simulink model "PubIfDecisionTOS_MDL"  (R2020b)
settings: configuration reference "DspaceConfig" (kept outside this file)
PostLoadFcn:
  | if any(exist('dsrtsu_mdlpostloadfcn', 'file') ~= 0), dsrtsu_mdlpostloadfcn('Execute', bdroot); end
InitFcn:
  | , if any(exist('dsmpb_private', 'file') ~= 0), dsmpb_private('dsmpb_mdlclblib', 'Init', bdroot); end,
undefined symbols (not defined in the file or in its folder): C_TOS_ACCEgoRAxletoFbumplength_m, C_TOS_ACCTargetFront_Flag, C_TOS_AEBJAPedObjDxThre_Val, C_TOS_AEBJAPedObjDyThre_Val, C_TOS_AEBJATargetSize_Val, C_TOS_AEBJAVehObjDxThre_Val, C_TOS_AEBJAVehObjDyThre_Val, C_TOS_AEBJuncPedTargetSize_Val, C_TOS_AEBLatObjDxThre_Val, C_TOS_AEBLatPedDyThre_Val, C_TOS_AEBLatTargetSize_Val, C_TOS_AEBLongTargetInEgoFront_Flag, C_TOS_axAbsGround_Parameter, C_TOS_CameraConfirmedFlag, C_TOS_CNsubjWidth, C_TOS_CurrentLaneCoreMinWidth_Val, C_TOS_CutInProb_Val_Zero, C_TOS_CutOutProb_Val_Zero, C_TOS_D2R_Val, C_TOS_DefaultValueObjectToCenterLine_dy, C_TOS_EgoCarWidth_Val, C_TOS_EgoDxRefPoint_m, C_TOS_EgoRAxletoFbumplength_m, C_TOS_HalfWidthVehicle_Con, C_TOS_HWA_CurrentLaneFlag, C_TOS_HWA_LeftLaneFlag, C_TOS_HWA_MovingDir_Vaild, C_TOS_HWA_MovState_Vaild, C_TOS_HWA_RightLaneFlag, C_TOS_LaneLineCourseErrorFront, C_TOS_LaneLineCourseErrorRear, C_TOS_MotorbikeDefaultWidth_m, C_TOS_NumberOfEffectiveTargets, C_TOS_Obj_Age_Val, C_TOS_Objdx_Constraint_Val, C_TOS_ObjectDefaultWidth_m, C_TOS_ObjInCurrentLane_Val, C_TOS_ObjInCurrentLaneValid, C_TOS_ObjInLeftLaneValid, C_TOS_ObjInRightLaneValid, C_TOS_ObjNotInCurrentLane_Val, C_TOS_ObjNotREElementType, C_TOS_ObjPredictDis_dy_ConstantVal_Zeros, C_TOS_ObjToCenterLine_ConstantVal_Zeros, C_TOS_OFMObjIDInvilad_Val, C_TOS_PIL_LatDisCons_Val_zero, C_TOS_PIL_ObjectCutInFlag_b, C_TOS_PIL_ObjectCutOutFlag_b, C_TOS_PIL_ObjLaneProb_al_Val, C_TOS_PP_ObjFusType_FC_Confirm_b, C_TOS_PP_ObjFusType_FC_FR_Confirm_b, C_TOS_PP_ObjFusType_FR_Confirm_b, C_TOS_RE_80BoolDefault_Val, C_TOS_RE_80Single181Default_Val, C_TOS_RE_80Single255Default_Val, C_TOS_RE_80Uint8Default_Val, C_TOS_RE_D2R, C_TOS_RE_D_180_Val, C_TOS_RE_InvalidObjectID_Val, C_TOS_RE_InvalidTargetChainDir_Val ... (+142)
libraries: simulink x1650, TOS_LIB x361, canfdmsglib x14
(part 9 of 69)

== system PubIfDecisionTOS_MDL/TOS_20201112/TOS_2012080320/PIL_1029/BoundaryCalculat/ObjectToCenterLine_dyc/RightLane ==
  CenterOfRightLane : Inport
  OFM_SignalVerification : Inport  Port=2
  Bus Selector : BusSelector  OutputSignals=TOS_OFMObjValid_Flag,Object_ID,Object_Age
  Bus Selector3 : BusSelector  OutputSignals=CenterLine01.PC0,CenterLine01.PC1,CenterLine01.PC2,CenterLine01.PC3,CenterLine01.dDisStart,CenterLine01.dDisEnd,CenterLine02.PC0,CenterLine02.PC1,CenterLine02.PC2,CenterLine02.PC3,CenterLine02.dDisStart,CenterLine02.dDisEnd,CenterLine03.PC0,CenterLine03.PC1,CenterLine03.PC2,CenterLine03.PC3,CenterLine03.dDisStart,CenterLine03.dDisEnd,CenterLine04.PC0,CenterLine04.PC1,CenterLine04.PC2,CenterLine04.PC3,CenterLine04.dDisStart,CenterLine04.dDisEnd,CenterLine05.PC0,CenterLine05.PC1,CenterLine05.PC2,CenterLine05.PC3,CenterLine05.dDisStart,CenterLine05.dDisEnd,CenterLine06.PC0,CenterLine06.PC1,CenterLine06.PC2,CenterLine06.PC3,CenterLine06.dDisStart,CenterLine06.dDisEnd
  Bus Selector4 : BusSelector  OutputSignals=TOS_OFMObjValid_Flag,Object_DY,Object_DX
  PIL_ObjectToCenterLine_dy_Filt : Subsystem
  RightCenterLine_dyc : Subsystem
  PIL_RightCenterLine_dyc : Outport
  PIL_RightCenterLine_dyc_Filt : Outport  Port=2
  wires:
  OFM_SignalVerification/1 -> [OFM_SignalVerification], Bus Selector4/1
  CenterOfRightLane/1 -> Bus Selector3/1
  Bus Selector3/34 -> RightCenterLine_dyc/37(line06_C3)  "<PC3>"
  Bus Selector3/35 -> RightCenterLine_dyc/38(line06_dDisStart)  "<dDisStart>"
  Bus Selector3/25 -> RightCenterLine_dyc/28(line05_C0)  "<PC0>"
  Bus Selector3/9 -> RightCenterLine_dyc/12(line02_C2)  "<PC2>"
  Bus Selector3/6 -> RightCenterLine_dyc/9(line01_dDisEnd)  "<dDisEnd>"
  Bus Selector3/22 -> RightCenterLine_dyc/25(line04_C3)  "<PC3>"
  Bus Selector3/31 -> RightCenterLine_dyc/34(line06_C0)  "<PC0>"
  Bus Selector3/16 -> RightCenterLine_dyc/19(line03_C3)  "<PC3>"
  Bus Selector3/8 -> RightCenterLine_dyc/11(line02_C1)  "<PC1>"
  Bus Selector4/1 -> RightCenterLine_dyc/1(TOS_OFMObjValid_Flag)  "<TOS_OFMObjValid_Flag>"
  Bus Selector3/33 -> RightCenterLine_dyc/36(line06_C2)  "<PC2>"
  Bus Selector3/10 -> RightCenterLine_dyc/13(line02_C3)  "<PC3>"
  Bus Selector3/14 -> RightCenterLine_dyc/17(line03_C1)  "<PC1>"
  Bus Selector3/1 -> RightCenterLine_dyc/4(line01_C0)  "<PC0>"
  Bus Selector3/28 -> RightCenterLine_dyc/31(line05_C3)  "<PC3>"
  Bus Selector3/32 -> RightCenterLine_dyc/35(line06_C1)  "<PC1>"
  Bus Selector3/27 -> RightCenterLine_dyc/30(line05_C2)  "<PC2>"
  Bus Selector3/20 -> RightCenterLine_dyc/23(line04_C1)  "<PC1>"
  Bus Selector3/30 -> RightCenterLine_dyc/33(line05_dDisEnd)  "<dDisEnd>"
  Bus Selector3/21 -> RightCenterLine_dyc/24(line04_C2)  "<PC2>"
  Bus Selector3/17 -> RightCenterLine_dyc/20(line03_dDisStart)  "<dDisStart>"
  Bus Selector3/26 -> RightCenterLine_dyc/29(line05_C1)  "<PC1>"
  Bus Selector3/11 -> RightCenterLine_dyc/14(line02_dDisStart)  "<dDisStart>"
  Bus Selector3/29 -> RightCenterLine_dyc/32(line05_dDisStart)  "<dDisStart>"
  Bus Selector3/24 -> RightCenterLine_dyc/27(line04_dDisEnd)  "<dDisEnd>"
  Bus Selector3/15 -> RightCenterLine_dyc/18(line03_C2)  "<PC2>"
  Bus Selector3/23 -> RightCenterLine_dyc/26(line04_dDisStart)  "<dDisStart>"
  Bus Selector4/2 -> RightCenterLine_dyc/2(Object_DY)  "<Object_DY>"
  Bus Selector3/13 -> RightCenterLine_dyc/16(line03_C0)  "<PC0>"
  Bus Selector3/19 -> RightCenterLine_dyc/22(line04_C0)  "<PC0>"
  Bus Selector3/36 -> RightCenterLine_dyc/39(line06_dDisEnd)  "<dDisEnd>"
  Bus Selector3/18 -> RightCenterLine_dyc/21(line03_dDisEnd)  "<dDisEnd>"
  Bus Selector3/12 -> RightCenterLine_dyc/15(line02_dDisEnd)  "<dDisEnd>"
  Bus Selector4/3 -> RightCenterLine_dyc/3(Object_DX)  "<Object_DX>"
  Bus Selector3/5 -> RightCenterLine_dyc/8(line01_dDisStart)  "<dDisStart>"
  Bus Selector3/7 -> RightCenterLine_dyc/10(line02_C0)  "<PC0>"
  Bus Selector3/4 -> RightCenterLine_dyc/7(line01_C3)  "<PC3>"
  Bus Selector3/3 -> RightCenterLine_dyc/6(line01_C2)  "<PC2>"
  Bus Selector3/2 -> RightCenterLine_dyc/5(line01_C1)  "<PC1>"
  Bus Selector/2 -> PIL_ObjectToCenterLine_dy_Filt/2(Object_ID)  "<Object_ID>"
  RightCenterLine_dyc/1(ObjectToCenterLine_dyc_RightLane) -> PIL_RightCenterLine_dyc/1, PIL_ObjectToCenterLine_dy_Filt/4(ObjectToCenterLine_dy)
  PIL_ObjectToCenterLine_dy_Filt/1(PIL_ObjectToCenterLine_dy_Filt) -> PIL_RightCenterLine_dyc_Filt/1
  Bus Selector/1 -> PIL_ObjectToCenterLine_dy_Filt/1(TOS_OFMObjValid_Flag)  "<TOS_OFMObjValid_Flag>"
  Bus Selector/3 -> PIL_ObjectToCenterLine_dy_Filt/3(Object_Age)  "<Object_Age>"
  [OFM_SignalVerification] -> Bus Selector/1

== system PubIfDecisionTOS_MDL/TOS_20201112/TOS_2012080320/PIL_1029/BoundaryCalculat/ObjectToCenterLine_dyc/SameLane ==
  Same_CenterLine : Inport
  OFM_SignalVerification : Inport  Port=2
  Bus Selector : BusSelector  OutputSignals=TOS_OFMObjValid_Flag,Object_ID,Object_Age
  Bus Selector3 : BusSelector  OutputSignals=CenterLine01.PC0,CenterLine01.PC1,CenterLine01.PC2,CenterLine01.PC3,CenterLine01.dDisStart,CenterLine01.dDisEnd,CenterLine02.PC0,CenterLine02.PC1,CenterLine02.PC2,CenterLine02.PC3,CenterLine02.dDisStart,CenterLine02.dDisEnd,CenterLine03.PC0,CenterLine03.PC1,CenterLine03.PC2,CenterLine03.PC3,CenterLine03.dDisStart,CenterLine03.dDisEnd,CenterLine04.PC0,CenterLine04.PC1,CenterLine04.PC2,CenterLine04.PC3,CenterLine04.dDisStart,CenterLine04.dDisEnd,CenterLine05.PC0,CenterLine05.PC1,CenterLine05.PC2,CenterLine05.PC3,CenterLine05.dDisStart,CenterLine05.dDisEnd,CenterLine06.PC0,CenterLine06.PC1,CenterLine06.PC2,CenterLine06.PC3,CenterLine06.dDisStart,CenterLine06.dDisEnd
  Bus Selector4 : BusSelector  OutputSignals=TOS_OFMObjValid_Flag,Object_DY,Object_DX
  PIL_ObjectToCenterLine_dy_Filt : Subsystem
  SameCenterLine_dyc : Subsystem
  PIL_SameCenterLine_dyc : Outport
  PIL_SameCenterLine_dyc_Filt : Outport  Port=2
  wires:
  Bus Selector3/2 -> SameCenterLine_dyc/5(line01_C1)  "<PC1>"
  Bus Selector3/3 -> SameCenterLine_dyc/6(line01_C2)  "<PC2>"
  Bus Selector3/4 -> SameCenterLine_dyc/7(line01_C3)  "<PC3>"
  Bus Selector3/7 -> SameCenterLine_dyc/10(line02_C0)  "<PC0>"
  Bus Selector3/5 -> SameCenterLine_dyc/8(line01_dDisStart)  "<dDisStart>"
  Bus Selector4/3 -> SameCenterLine_dyc/3(Object_DX)  "<Object_DX>"
  Bus Selector3/12 -> SameCenterLine_dyc/15(line02_dDisEnd)  "<dDisEnd>"
  Bus Selector3/18 -> SameCenterLine_dyc/21(line03_dDisEnd)  "<dDisEnd>"
  Bus Selector3/36 -> SameCenterLine_dyc/39(line06_dDisEnd)  "<dDisEnd>"
  Bus Selector3/19 -> SameCenterLine_dyc/22(line04_C0)  "<PC0>"
  Bus Selector3/13 -> SameCenterLine_dyc/16(line03_C0)  "<PC0>"
  Bus Selector4/2 -> SameCenterLine_dyc/2(Object_DY)  "<Object_DY>"
  Bus Selector3/23 -> SameCenterLine_dyc/26(line04_dDisStart)  "<dDisStart>"
  Bus Selector3/15 -> SameCenterLine_dyc/18(line03_C2)  "<PC2>"
  Bus Selector3/24 -> SameCenterLine_dyc/27(line04_dDisEnd)  "<dDisEnd>"
  Bus Selector3/29 -> SameCenterLine_dyc/32(line05_dDisStart)  "<dDisStart>"
  Bus Selector3/11 -> SameCenterLine_dyc/14(line02_dDisStart)  "<dDisStart>"
  Bus Selector3/26 -> SameCenterLine_dyc/29(line05_C1)  "<PC1>"
  Bus Selector3/17 -> SameCenterLine_dyc/20(line03_dDisStart)  "<dDisStart>"
  Bus Selector3/21 -> SameCenterLine_dyc/24(line04_C2)  "<PC2>"
  Bus Selector3/30 -> SameCenterLine_dyc/33(line05_dDisEnd)  "<dDisEnd>"
  Bus Selector3/20 -> SameCenterLine_dyc/23(line04_C1)  "<PC1>"
  Bus Selector3/27 -> SameCenterLine_dyc/30(line05_C2)  "<PC2>"
  Bus Selector3/32 -> SameCenterLine_dyc/35(line06_C1)  "<PC1>"
  Bus Selector3/28 -> SameCenterLine_dyc/31(line05_C3)  "<PC3>"
  Bus Selector3/1 -> SameCenterLine_dyc/4(line01_C0)  "<PC0>"
  Bus Selector3/14 -> SameCenterLine_dyc/17(line03_C1)  "<PC1>"
  Bus Selector3/10 -> SameCenterLine_dyc/13(line02_C3)  "<PC3>"
  Bus Selector3/33 -> SameCenterLine_dyc/36(line06_C2)  "<PC2>"
  Bus Selector4/1 -> SameCenterLine_dyc/1(TOS_OFMObjValid_Flag)  "<TOS_OFMObjValid_Flag>"
  Bus Selector3/8 -> SameCenterLine_dyc/11(line02_C1)  "<PC1>"
  Bus Selector3/16 -> SameCenterLine_dyc/19(line03_C3)  "<PC3>"
  Bus Selector3/31 -> SameCenterLine_dyc/34(line06_C0)  "<PC0>"
  Bus Selector3/22 -> SameCenterLine_dyc/25(line04_C3)  "<PC3>"
  Bus Selector3/6 -> SameCenterLine_dyc/9(line01_dDisEnd)  "<dDisEnd>"
  Bus Selector3/9 -> SameCenterLine_dyc/12(line02_C2)  "<PC2>"
  Bus Selector3/25 -> SameCenterLine_dyc/28(line05_C0)  "<PC0>"
  Bus Selector3/35 -> SameCenterLine_dyc/38(line06_dDisStart)  "<dDisStart>"
  Bus Selector3/34 -> SameCenterLine_dyc/37(line06_C3)  "<PC3>"
  Same_CenterLine/1 -> Bus Selector3/1
  OFM_SignalVerification/1 -> [OFM_SignalVerification], Bus Selector4/1
  Bus Selector/2 -> PIL_ObjectToCenterLine_dy_Filt/2(Object_ID)  "<Object_ID>"
  SameCenterLine_dyc/1(SameCenterLine_dyc) -> PIL_SameCenterLine_dyc/1, PIL_ObjectToCenterLine_dy_Filt/4(ObjectToCenterLine_dy)
  PIL_ObjectToCenterLine_dy_Filt/1(PIL_ObjectToCenterLine_dy_Filt) -> PIL_SameCenterLine_dyc_Filt/1
  Bus Selector/1 -> PIL_ObjectToCenterLine_dy_Filt/1(TOS_OFMObjValid_Flag)  "<TOS_OFMObjValid_Flag>"
  Bus Selector/3 -> PIL_ObjectToCenterLine_dy_Filt/3(Object_Age)  "<Object_Age>"
  [OFM_SignalVerification] -> Bus Selector/1

== system PubIfDecisionTOS_MDL/TOS_20201112/TOS_2012080320/PIL_1029/ObjCutInOut_Prob/ObjectCutIn/CutInProb_Calculate ==
  TOS_OFMObjValid_Flag : Inport  Partition=on  PartitionDimension=1  PartitionWidth=1  PartitionOffset=0
  Object_Width : Inport  Port=2  OutDataTypeStr=single  Partition=on  PartitionDimension=1  PartitionWidth=1  PartitionOffset=0
  Object_DX : Inport  Port=3  OutDataTypeStr=single  Partition=on  PartitionDimension=1  PartitionWidth=1  PartitionOffset=0
  Object_DY : Inport  Port=4  OutDataTypeStr=single  Partition=on  PartitionDimension=1  PartitionWidth=1  PartitionOffset=0
  Object_Age : Inport  Port=5  OutDataTypeStr=uint16  Partition=on  PartitionDimension=1  PartitionWidth=1  PartitionOffset=0
  Object_Type : Inport  Port=6  Partition=on  PartitionDimension=1  PartitionWidth=1  PartitionOffset=0
  PP_ObjectToCenterLine_dy : Inport  Port=7  OutDataTypeStr=single  Partition=on  PartitionDimension=1  PartitionWidth=1  PartitionOffset=0
  PP_ObjectToCenterLine_vyc : Inport  Port=8  OutDataTypeStr=single  Partition=on  PartitionDimension=1  PartitionWidth=1  PartitionOffset=0
  PIL_ObjectToCenterLine_dy_Filt : Inport  Port=9  OutDataTypeStr=single  Partition=on  PartitionDimension=1  PartitionWidth=1  PartitionOffset=0
  PP_CurrentLaneWidth : Inport  Port=10
  Compare To Constant : simulink/Logic and Bit Operations/Compare To Constant  relop===  const=C_TOS_OFMObjIDInvilad_Val  OutDataTypeStr=boolean
      settings: AttributesFormatString=C_TOS_OFMObjIDInvilad_Val = 0
  CutInProb_CalculateDefault : Subsystem  TreatAsAtomicUnit=on
  CutInProb_Calculate_ : Subsystem
  For Each : ForEach  DisableCoverage=on
  If : If  IfExpression=u1 ~= 0
  Merge{,1..4} (5 alike) : Merge
  PIL_CutInPredictTime_ObserVale : Outport  OutDataTypeStr=single  ConcatenationDimension=1
  PIL_CutInPredictTime_dxConstraint_ObserVale : Outport  Port=2  OutDataTypeStr=single  ConcatenationDimension=1
  PIL_CutInPredictDis_dy_ObjWidthConstraint_ObserVale : Outport  Port=3  ConcatenationDimension=1
  PIL_ObjectCutinMindFlg_ObserVale : Outport  Port=4  OutDataTypeStr=boolean  ConcatenationDimension=1
  CutInProb_Calculate : Outport  Port=5  ConcatenationDimension=1
  wires:
  Object_Width/1 -> CutInProb_Calculate_/1(Object_Width)  "Object_Width"
  Object_DX/1 -> CutInProb_Calculate_/2(Object_DX)  "Object_DX"
  Object_DY/1 -> CutInProb_Calculate_/3(Object_DY)  "Object_DY"
  Object_Age/1 -> CutInProb_Calculate_/4(Object_Age)  "Object_Age"
  Object_Type/1 -> CutInProb_Calculate_/5(Object_Type)  "Object_Type"
  PP_ObjectToCenterLine_dy/1 -> CutInProb_Calculate_/6(PP_ObjectToCenterLine_dy)  "PP_ObjectToCenterLine_dy"
  PP_ObjectToCenterLine_vyc/1 -> CutInProb_Calculate_/7(PP_ObjectToCenterLine_vyc)  "PP_ObjectToCenterLine_vyc"
  PIL_ObjectToCenterLine_dy_Filt/1 -> CutInProb_Calculate_/8(PIL_ObjectToCenterLine_dy_Filt)  "PIL_ObjectToCenterLine_dy_Filt"
  PP_CurrentLaneWidth/1 -> CutInProb_Calculate_/9(PP_CurrentLaneWidth)  "CurrentLaneWidth"
  TOS_OFMObjValid_Flag/1 -> Compare To Constant/1
  If/2 -> CutInProb_Calculate_/Action
  Compare To Constant/1 -> If/1
  If/1 -> CutInProb_CalculateDefault/Action
  CutInProb_Calculate_/1(PIL_CutInPredictTime_ObserVale) -> Merge/2
  CutInProb_Calculate_/2(PIL_CutInPredictTime_dxConstraint_ObserVale) -> Merge1/2
  CutInProb_Calculate_/3(PIL_CutInPredictDis_dy_ObjWidthConstraint_ObserVale) -> Merge2/2
  CutInProb_Calculate_/4(PIL_ObjectCutinMindFlg_ObserVale) -> Merge3/2
  CutInProb_Calculate_/5(CutInProb_Calculate) -> Merge4/2
  CutInProb_CalculateDefault/1(PIL_CutInPredictTime_ObserVale) -> Merge/1
  CutInProb_CalculateDefault/2(PIL_CutInPredictTime_dxConstraint_ObserVale) -> Merge1/1
  CutInProb_CalculateDefault/3(PIL_CutInPredictDis_dy_ObjWidthConstraint_ObserVale) -> Merge2/1
  CutInProb_CalculateDefault/4(PIL_ObjectCutinMindFlg_ObserVale) -> Merge3/1
  CutInProb_CalculateDefault/5(CutInProb_Calculate) -> Merge4/1
  Merge/1 -> PIL_CutInPredictTime_ObserVale/1
  Merge1/1 -> PIL_CutInPredictTime_dxConstraint_ObserVale/1
  Merge2/1 -> PIL_CutInPredictDis_dy_ObjWidthConstraint_ObserVale/1
  Merge3/1 -> PIL_ObjectCutinMindFlg_ObserVale/1
  Merge4/1 -> CutInProb_Calculate/1

== system PubIfDecisionTOS_MDL/TOS_20201112/TOS_2012080320/PIL_1029/ObjCutInOut_Prob/ObjectCutIn/CutInProb_Pluse ==
  CutInProb_Pluse_K1 : Inport  OutDataTypeStr=single  Partition=on  PartitionDimension=1  PartitionWidth=1  PartitionOffset=0
  CutInProb_ScopeConstraint : Inport  Port=2  OutDataTypeStr=single  Partition=on  PartitionDimension=1  PartitionWidth=1  PartitionOffset=0
  Object_Dx : Inport  Port=3  OutDataTypeStr=single  Partition=on  PartitionDimension=1  PartitionWidth=1  PartitionOffset=0
  TOS_OFMObjValid_Flag : Inport  Port=4  Partition=on  PartitionDimension=1  PartitionWidth=1  PartitionOffset=0
  Object_MovingState : Inport  Port=5  Partition=on  PartitionDimension=1  PartitionWidth=1  PartitionOffset=0
  Compare To Constant1 : simulink/Logic and Bit Operations/Compare To Constant  relop=~=  const=C_TOS_OFMObjIDInvilad_Val  OutDataTypeStr=boolean
      settings: AttributesFormatString=C_TOS_OFMObjIDInvilad_Val = 0
  Compare To Constant6 : simulink/Logic and Bit Operations/Compare To Constant  relop===  const=OFM_OBJ_MOVINGSTATE_E.MOVING  OutDataTypeStr=boolean
      settings: AttributesFormatString=OFM_OBJ_MOVINGSTATE_E.MOVING = 2
  CutInProb_Pluse : Subsystem
  CutInProb_PluseDefault : Subsystem  TreatAsAtomicUnit=on
  Data Type Conversion1 : DataTypeConversion  OutDataTypeStr=Enum: OFM_OBJ_MOVINGSTATE_E
  For Each : ForEach  DisableCoverage=on
  If1 : If  IfExpression=u1 == 1
  Logical Operator2 : Logic  AllPortsSameDT=off  OutDataTypeStr=boolean
  Merge : Merge
  Merge1 : Merge
  PIL_CutInProb_Pluse : Outport  OutDataTypeStr=single  ConcatenationDimension=1
  PIL_ObjectCutInFlag : Outport  Port=2  ConcatenationDimension=1
  wires:
  CutInProb_Pluse/2(PIL_ObjectCutInFlag) -> Merge1/1
  CutInProb_Pluse/1(PIL_CutInProb_Pluse) -> Merge/1
  CutInProb_PluseDefault/2(PIL_ObjectCutInFlag) -> Merge1/2
  CutInProb_PluseDefault/1(PIL_CutInProb_Pluse) -> Merge/2
  Data Type Conversion1/1 -> Compare To Constant6/1
  Compare To Constant6/1 -> Logical Operator2/2
  TOS_OFMObjValid_Flag/1 -> Compare To Constant1/1
  Object_MovingState/1 -> Data Type Conversion1/1
  Logical Operator2/1 -> If1/1
  Compare To Constant1/1 -> Logical Operator2/1
  CutInProb_Pluse_K1/1 -> CutInProb_Pluse/1(CutInProb_Pluse_K1)
  CutInProb_ScopeConstraint/1 -> CutInProb_Pluse/2(CutInProb_ScopeConstraint)
  Object_Dx/1 -> CutInProb_Pluse/3(Object_Dx)
  If1/2 -> CutInProb_PluseDefault/Action
  If1/1 -> CutInProb_Pluse/Action
  Merge/1 -> PIL_CutInProb_Pluse/1
  Merge1/1 -> PIL_ObjectCutInFlag/1

== system PubIfDecisionTOS_MDL/TOS_20201112/TOS_2012080320/PIL_1029/ObjCutInOut_Prob/ObjectCutOut/CutOutProb_Calculate ==
  TOS_OFMObjValid_Flag : Inport  Partition=on  PartitionDimension=1  PartitionWidth=1  PartitionOffset=0
  Object_Width : Inport  Port=2  Partition=on  PartitionDimension=1  PartitionWidth=1  PartitionOffset=0
  Object_DX : Inport  Port=3  Partition=on  PartitionDimension=1  PartitionWidth=1  PartitionOffset=0
  Object_DY : Inport  Port=4  Partition=on  PartitionDimension=1  PartitionWidth=1  PartitionOffset=0
  Object_Age : Inport  Port=5  Partition=on  PartitionDimension=1  PartitionWidth=1  PartitionOffset=0
  Object_Type : Inport  Port=6  Partition=on  PartitionDimension=1  PartitionWidth=1  PartitionOffset=0
  PP_ObjectToCenterLine_dy : Inport  Port=7  Partition=on  PartitionDimension=1  PartitionWidth=1  PartitionOffset=0
  PP_ObjectToCenterLine_vyc : Inport  Port=8  Partition=on  PartitionDimension=1  PartitionWidth=1  PartitionOffset=0
  PIL_ObjectToCenterLine_dy_Filt : Inport  Port=9  Partition=on  PartitionDimension=1  PartitionWidth=1  PartitionOffset=0
  Object_VY : Inport  Port=10  Partition=on  PartitionDimension=1  PartitionWidth=1  PartitionOffset=0
  Compare To Constant : simulink/Logic and Bit Operations/Compare To Constant  relop===  const=C_TOS_OFMObjIDInvilad_Val  OutDataTypeStr=boolean
      settings: AttributesFormatString=C_TOS_OFMObjIDInvilad_Val = 0
  CutOutProb_Calculate : Subsystem
  CutOutProb_CalculateDefault : Subsystem  TreatAsAtomicUnit=on
  For Each : ForEach  DisableCoverage=on
  If : If  IfExpression=u1 ~= 0
  Merge{,1..7} (8 alike) : Merge
  PIL_CutOutPredictTime_ObserVale : Outport  OutDataTypeStr=single  ConcatenationDimension=1
  PIL_CutOutPredictTime_dxConstraint_ObserVale : Outport  Port=2  OutDataTypeStr=single  ConcatenationDimension=1
  PIL_CutOutPredictDis_dy_ObjWidthConstraint_ObserVale : Outport  Port=3  ConcatenationDimension=1
  PIL_ObjectCutOutMindFlg_ObserVale : Outport  Port=4  OutDataTypeStr=boolean  ConcatenationDimension=1
  PIL_ObjectCutoutMindFlg1_ObserVale : Outport  Port=5  OutDataTypeStr=boolean  ConcatenationDimension=1
  PIL_ObjectCutoutMindFlg2_ObserVale : Outport  Port=6  OutDataTypeStr=boolean  ConcatenationDimension=1
  PIL_ObjectCutoutMindFlg3_ObserVale : Outport  Port=7  OutDataTypeStr=boolean  ConcatenationDimension=1
  PIL_CutOutProb_ScopeConstraint : Outport  Port=8  ConcatenationDimension=1
  wires:
  Object_VY/1 -> CutOutProb_Calculate/9(Object_VY)
  Object_Width/1 -> CutOutProb_Calculate/1(Object_Width)
  If/2 -> CutOutProb_Calculate/Action
  CutOutProb_Calculate/1(PIL_CutOutPredictTime_ObserVale) -> Merge/2
  TOS_OFMObjValid_Flag/1 -> Compare To Constant/1
  Compare To Constant/1 -> If/1
  Object_DX/1 -> CutOutProb_Calculate/2(Object_DX)
  PP_ObjectToCenterLine_dy/1 -> CutOutProb_Calculate/6(PP_ObjectToCenterLine_dy)
  Object_Type/1 -> CutOutProb_Calculate/5(Object_Type)
  Object_Age/1 -> CutOutProb_Calculate/4(Object_Age)
  Object_DY/1 -> CutOutProb_Calculate/3(Object_DY)
  PP_ObjectToCenterLine_vyc/1 -> CutOutProb_Calculate/7(PP_ObjectToCenterLine_vyc)
  CutOutProb_Calculate/4(PIL_ObjectCutOutMindFlg_ObserVale) -> Merge3/2
  CutOutProb_Calculate/2(PIL_CutOutPredictTime_dxConstraint_ObserVale) -> Merge1/2
  CutOutProb_Calculate/3(PIL_CutOutPredictDis_dy_ObjWidthConstraint_ObserVale) -> Merge2/2
  PIL_ObjectToCenterLine_dy_Filt/1 -> CutOutProb_Calculate/8(PIL_ObjectToCenterLine_dy_Filt)
  CutOutProb_Calculate/5(PIL_CutOutProb_ScopeConstraint) -> Merge4/2
  If/1 -> CutOutProb_CalculateDefault/Action
  Merge/1 -> PIL_CutOutPredictTime_ObserVale/1
  CutOutProb_CalculateDefault/1(PIL_CutOutPredictTime_ObserVale) -> Merge/1
  CutOutProb_CalculateDefault/2(PIL_CutOutPredictTime_Constraint_ObserVale) -> Merge1/1
  Merge1/1 -> PIL_CutOutPredictTime_dxConstraint_ObserVale/1
  Merge2/1 -> PIL_CutOutPredictDis_dy_ObjWidthConstraint_ObserVale/1
  CutOutProb_CalculateDefault/3(PIL_CutOutPredictDis_dy_ObjWidthConstraint_ObserVale) -> Merge2/1
  CutOutProb_CalculateDefault/4(PIL_ObjectCutOutMindFlg_ObserVale) -> Merge3/1
  Merge3/1 -> PIL_ObjectCutOutMindFlg_ObserVale/1
  CutOutProb_CalculateDefault/5(PIL_CutOutProb_ScopeConstraint) -> Merge4/1
  Merge4/1 -> PIL_CutOutProb_ScopeConstraint/1
  CutOutProb_Calculate/6(PIL_ObjectCutoutMindFlg1_ObserVale) -> Merge5/2
  CutOutProb_Calculate/7(PIL_ObjectCutoutMindFlg2_ObserVale) -> Merge6/2
  CutOutProb_Calculate/8(PIL_ObjectCutoutMindFlg3_ObserVale) -> Merge7/2
  CutOutProb_CalculateDefault/6(PIL_ObjectCutoutMindFlg1_ObserVale) -> Merge5/1
  CutOutProb_CalculateDefault/7(PIL_ObjectCutoutMindFlg2_ObserVale) -> Merge6/1
  CutOutProb_CalculateDefault/8(PIL_ObjectCutoutMindFlg3_ObserVale) -> Merge7/1
  Merge5/1 -> PIL_ObjectCutoutMindFlg1_ObserVale/1
  Merge6/1 -> PIL_ObjectCutoutMindFlg2_ObserVale/1
  Merge7/1 -> PIL_ObjectCutoutMindFlg3_ObserVale/1

== system PubIfDecisionTOS_MDL/TOS_20201112/TOS_2012080320/PIL_1029/ObjCutInOut_Prob/ObjectCutOut/CutOutProb_Pluse ==
  CutOutProb_Pluse_K1 : Inport  OutDataTypeStr=single  Partition=on  PartitionDimension=1  PartitionWidth=1  PartitionOffset=0
  CutOutProb_ScopeConstraint : Inport  Port=2  OutDataTypeStr=single  Partition=on  PartitionDimension=1  PartitionWidth=1  PartitionOffset=0
  TOS_OFMObjValid_Flag : Inport  Port=3  Partition=on  PartitionDimension=1  PartitionWidth=1  PartitionOffset=0
  Object_MovingState : Inport  Port=4  Partition=on  PartitionDimension=1  PartitionWidth=1  PartitionOffset=0
  Compare To Constant : simulink/Logic and Bit Operations/Compare To Constant  relop=~=  const=C_TOS_OFMObjIDInvilad_Val  OutDataTypeStr=boolean
      settings: AttributesFormatString=C_TOS_OFMObjIDInvilad_Val = 0
  Compare To Constant6 : simulink/Logic and Bit Operations/Compare To Constant  relop===  const=OFM_OBJ_MOVINGSTATE_E.MOVING  OutDataTypeStr=boolean
      settings: AttributesFormatString=OFM_OBJ_MOVINGSTATE_E.MOVING = 2
  CutInProb_PluseDefault : Subsystem  TreatAsAtomicUnit=on
  Data Type Conversion1 : DataTypeConversion  OutDataTypeStr=Enum: OFM_OBJ_MOVINGSTATE_E
  For Each : ForEach  DisableCoverage=on
  If : If  IfExpression=u1 == 1
  Logical Operator2 : Logic  AllPortsSameDT=off  OutDataTypeStr=boolean
  Merge : Merge
  Merge1 : Merge
  Subsystem : Subsystem
  PIL_CutOutProb_Pluse : Outport  OutDataTypeStr=single  ConcatenationDimension=1
  PIL_ObjectCutOutFlag : Outport  Port=2  ConcatenationDimension=1
  wires:
  Logical Operator2/1 -> If/1
  Compare To Constant6/1 -> Logical Operator2/2
  Data Type Conversion1/1 -> Compare To Constant6/1
  Object_MovingState/1 -> Data Type Conversion1/1
  CutOutProb_Pluse_K1/1 -> Subsystem/1(CutOutProb_Pluse_K1)
  CutOutProb_ScopeConstraint/1 -> Subsystem/2(CutOutProb_ScopeConstraint)
  Subsystem/1(PIL_CutOutProb_Pluse) -> Merge/1
  Subsystem/2(PIL_ObjectCutOutFlag) -> Merge1/1
  If/1 -> Subsystem/Action
  Compare To Constant/1 -> Logical Operator2/1
  TOS_OFMObjValid_Flag/1 -> Compare To Constant/1
  If/2 -> CutInProb_PluseDefault/Action
  Merge/1 -> PIL_CutOutProb_Pluse/1
  CutInProb_PluseDefault/1(PIL_CutOutProb_Pluse) -> Merge/2
  Merge1/1 -> PIL_ObjectCutOutFlag/1
  CutInProb_PluseDefault/2(PIL_ObjectCutOutFlag) -> Merge1/2

== system PubIfDecisionTOS_MDL/TOS_20201112/TOS_2012080320/PIL_1029/ObjCutInOut_Prob/ObjectCutOut/Subsystem ==
  In1 : Inport  Partition=on  PartitionDimension=1  PartitionWidth=1  PartitionOffset=0
  For Each : ForEach  DisableCoverage=on
  Gain : Gain  Gain=0.33
  Sum of Elements : Sum  Inputs=+
  Tapped Delay : simulink/Discrete/Tapped Delay  vinit=0.0  samptime=-1  NumDelays=3  DelayOrder=Oldest  includeCurrent=off
  Out1 : Outport  ConcatenationDimension=1
  wires:
  Gain/1 -> Out1/1
  In1/1 -> Tapped Delay/1
  Tapped Delay/1 -> Sum of Elements/1
  Sum of Elements/1 -> Gain/1

== system PubIfDecisionTOS_MDL/TOS_20201112/TOS_2012080320/PIL_1029/OverlapRatio_Calculate/PIL_OverlapCalculation/OverlapRatioCalcFlow/overlapRatioCalc ==
  note: dyCriticalEgoObj - Abs(dyOverlapActual)
      | overlapRatio = -------------------------------------------------------------
      | 						dyCriticalEgoObj
  dyCriticalEgoObj : Inport
  dyOverlapActual : Inport  Port=2
  f : TriggerPort  TriggerType=function-call  VariantControl=Variant
      settings: CopyFcn=Stateflow.SLINSF.SimulinkMan.removeBlockPreDeleteFcn  PreDeleteFcn=Stateflow.SLINSF.SimulinkMan.unsafePredeleteFcn
  Abs2 : Abs
  Add1 : Sum  Inputs=+-
  Divide : Product  Inputs=*/
  overlapRatio : Outport
  wires:
  dyOverlapActual/1 -> Abs2/1
  dyCriticalEgoObj/1 -> Divide/2, Add1/1
  Divide/1 -> overlapRatio/1
  Abs2/1 -> Add1/2
  Add1/1 -> Divide/1

== system PubIfDecisionTOS_MDL/TOS_20201112/TOS_2012080320/PIL_1029/OverlapRatio_Calculate/PIL_OverlapCalculation/TargetWidthCalc ==
  ObjectWidth : Inport
  ObjectTypeCameraConfirmed : Inport  Port=2
  object_MovingState : Inport  Port=3
  Object_Type : Inport  Port=4
  Add : Sum
  Compare To Constant : simulink/Logic and Bit Operations/Compare To Constant  relop===  const=OFM_OBJ_MOVINGSTATE_E.MOVING  OutDataTypeStr=boolean
      settings: AttributesFormatString=OFM_OBJ_MOVINGSTATE_E.MOVING = 2
  Compare To Constant1 : simulink/Logic and Bit Operations/Compare To Constant  relop===  const=OFM_OBJ_TYPE_E.CAR  OutDataTypeStr=boolean
      settings: AttributesFormatString=OFM_OBJ_TYPE_E.CAR = 2
  Compare To Constant2 : simulink/Logic and Bit Operations/Compare To Constant  relop===  const=C_TOS_CameraConfirmedFlag  OutDataTypeStr=boolean
      settings: AttributesFormatString=C_TOS_CameraConfirmedFlag = 1
  Compare To Constant3 : simulink/Logic and Bit Operations/Compare To Constant  relop===  const=OFM_OBJ_MOVINGSTATE_E.MOVING_SLOWLY  OutDataTypeStr=boolean
      settings: AttributesFormatString=OFM_OBJ_MOVINGSTATE_E.MOVING_SLOWLY = 5
  Compare To Constant4 : simulink/Logic and Bit Operations/Compare To Constant  relop===  const=OFM_OBJ_TYPE_E.TRUCK  OutDataTypeStr=boolean
      settings: AttributesFormatString=OFM_OBJ_TYPE_E.TRUCK = 3
  Compare To Constant5 : simulink/Logic and Bit Operations/Compare To Constant  relop===  const=OFM_OBJ_TYPE_E.MOTORBIKE  OutDataTypeStr=boolean
      settings: AttributesFormatString=OFM_OBJ_TYPE_E.MOTORBIKE = 4
  Compare To Constant6 : simulink/Logic and Bit Operations/Compare To Constant  relop===  const=OFM_OBJ_TYPE_E.BICYCLE  OutDataTypeStr=boolean
      settings: AttributesFormatString=OFM_OBJ_TYPE_E.BICYCLE = 5
  Compare To Constant7 : simulink/Logic and Bit Operations/Compare To Constant  relop===  const=OFM_OBJ_TYPE_E.PEDESTRIAN  OutDataTypeStr=boolean
      settings: AttributesFormatString=OFM_OBJ_TYPE_E.PEDESTRIAN = 6
  Constant : Constant  Value=P_TOS_ObjWidthThreshold_Overlap_Val
      settings: AttributesFormatString=P_TOS_ObjWidthThreshold_Overlap_Val = 0.4
  Data Type Conversion : DataTypeConversion  OutDataTypeStr=Enum: OFM_OBJ_TYPE_E
  Data Type Conversion1 : DataTypeConversion  OutDataTypeStr=Enum: OFM_OBJ_MOVINGSTATE_E
  Logical Operator1 : Logic  Operator=OR  AllPortsSameDT=off  OutDataTypeStr=boolean
  Logical Operator2 : Logic  Operator=OR  AllPortsSameDT=off  OutDataTypeStr=boolean
  Logical Operator3 : Logic  Operator=OR  AllPortsSameDT=off  OutDataTypeStr=boolean
  MovingObjWidth : Constant  Value=P_TOS_OverlapEgoWidthMO
      settings: AttributesFormatString=P_TOS_OverlapEgoWidthMO = 1
  Saturation : Saturate  UpperLimit=2.0  LowerLimit=1.2
  Saturation1 : Saturate  UpperLimit=0.8  LowerLimit=0.4
  Saturation2 : Saturate  LowerLimit=0.5
  StationaryObjWidth : Constant  Value=P_TOS_OverlapEgoWidthSO
      settings: AttributesFormatString=P_TOS_OverlapEgoWidthSO = 0.5
  Switch{,1..4} (5 alike) : Switch  Criteria=u2 ~= 0
  objWidth : Outport
  wires:
  Switch/1 -> objWidth/1
  StationaryObjWidth/1 -> Switch1/1
  Add/1 -> Switch/1
  Switch1/1 -> Switch/3
  Compare To Constant2/1 -> Switch/2
  ObjectTypeCameraConfirmed/1 -> Compare To Constant2/1
  Logical Operator3/1 -> Switch1/2
  MovingObjWidth/1 -> Switch1/3
  Compare To Constant3/1 -> Logical Operator3/2
  Compare To Constant/1 -> Logical Operator3/1
  Data Type Conversion1/1 -> Compare To Constant3/1, Compare To Constant/1
  object_MovingState/1 -> Data Type Conversion1/1
  Data Type Conversion/1 -> Compare To Constant7/1, Compare To Constant6/1, Compare To Constant5/1, Compare To Constant4/1, Compare To Constant1/1
  Object_Type/1 -> Data Type Conversion/1
  Constant/1 -> Add/2
  Compare To Constant1/1 -> Logical Operator1/1
  Compare To Constant4/1 -> Logical Operator1/2
  Compare To Constant5/1 -> Logical Operator2/1
  Compare To Constant6/1 -> Logical Operator2/2
  Logical Operator1/1 -> Switch2/2
  Saturation/1 -> Switch2/1
  Logical Operator2/1 -> Switch3/2
  ObjectWidth/1 -> Saturation1/1, Switch4/3, Saturation2/1, Saturation/1
  Saturation1/1 -> Switch3/1
  Switch3/1 -> Switch2/3
  Compare To Constant7/1 -> Switch4/2
  Saturation2/1 -> Switch4/1
  Switch4/1 -> Switch3/3
  Switch2/1 -> Add/1

== system PubIfDecisionTOS_MDL/TOS_20201112/TOS_2012080320/PIL_1029/OverlapRatio_Calculate/PIL_OverlapCalculation/dyCriticalEgoObjCalc ==
  note: 1.8
  objWidth : Inport
  Add : Sum
  Constant : Constant  Value=C_TOS_CNsubjWidth
  Gain1 : Gain  Gain=0.5
  Gain2 : Gain  Gain=0.5
  dyCriticalEgoObj : Outport
  wires:
  Gain2/1 -> Add/2
  Gain1/1 -> Add/1
  Add/1 -> dyCriticalEgoObj/1  "dyCriticalEgoObj"
  Constant/1 -> Gain2/1
  objWidth/1 -> Gain1/1

== system PubIfDecisionTOS_MDL/TOS_20201112/TOS_2012080320/PIL_1029/PIL_ObjectToCenterLine_dy_Filt/PIL_ObjectToCenterLine_dy/PP_SignalProcessingDefault ==
  Action Port : ActionPort  ActionPortLabel=if(u1 ~= 0)
  Constant : Constant  Value=0  OutDataTypeStr=uint8
  Constant1 : Constant  Value=255  OutDataTypeStr=single
  Obj_ID : Outport
  ObjectToCenterLine_dy_Filt : Outport  Port=2  OutDataTypeStr=single
  wires:
  Constant1/1 -> ObjectToCenterLine_dy_Filt/1
  Constant/1 -> Obj_ID/1

== system PubIfDecisionTOS_MDL/TOS_20201112/TOS_2012080320/PIL_1029/PIL_ObjectToCenterLine_dy_Filt/PIL_ObjectToCenterLine_dy/Subsystem ==
  ObjectID_Filt_K1 : Inport
  ObjectToCenterLine_dy_Filt_K1 : Inport  Port=2  OutDataTypeStr=single
  ObjectToCenterLine_dy : Inport  Port=3  OutDataTypeStr=single
  Object_ID : Inport  Port=4  OutDataTypeStr=uint8
  Object_Age : Inport  Port=5
  TOS_OFMObjValid_Flag : Inport  Port=6
  Action Port : ActionPort  ActionPortLabel=else
  Constant1 : Constant  Value=C_TOS_NumberOfEffectiveTargets  OutDataTypeStr=int32
      settings: AttributesFormatString=C_TOS_NumberOfEffectiveTargets = 80
  Constant2 : Constant  Value=P_TOS_PIL_ObjectToCenterLine_dy_CutInDeclineLimit  OutDataTypeStr=single
      settings: AttributesFormatString=P_TOS_PIL_ObjectToCenterLine_dy_CutInDeclineLimit = 0.1
  Constant8 : Constant  Value=P_TOS_PIL_ObjectToCenterLine_dy_CutInUpperLimit  OutDataTypeStr=single
      settings: AttributesFormatString=P_TOS_PIL_ObjectToCenterLine_dy_CutInUpperLimit = 0.5
  ObjectToCenterLine_dyFilit : MATLAB Function  TreatAsAtomicUnit=on
  Terminator : Terminator
  Obj_ID : Outport
  ObjectToCenterLine_dy_Filt : Outport  Port=2  OutDataTypeStr=single
  wires:
  TOS_OFMObjValid_Flag/1 -> ObjectToCenterLine_dyFilit/5(TOS_OFMObjValid_Flag)
  Object_Age/1 -> Terminator/1
  ObjectToCenterLine_dy_Filt_K1/1 -> ObjectToCenterLine_dyFilit/2(ObjectToCenterLine_dy_Filt_K1)
  Object_ID/1 -> Obj_ID/1, ObjectToCenterLine_dyFilit/4(Object_ID)
  ObjectID_Filt_K1/1 -> ObjectToCenterLine_dyFilit/1(ObjectID_Filt_K1)
  Constant2/1 -> ObjectToCenterLine_dyFilit/7(P_TOS_PIL_ObjectToCenterLine_dy_CutInDeclineLimit)
  Constant1/1 -> ObjectToCenterLine_dyFilit/8(Iterator_Num)
  ObjectToCenterLine_dy/1 -> ObjectToCenterLine_dyFilit/3(ObjectToCenterLine_dy)
  Constant8/1 -> ObjectToCenterLine_dyFilit/6(P_TOS_PIL_ObjectToCenterLine_dy_CutInUpperLimit)
  ObjectToCenterLine_dyFilit/1(ObjectToCenterLine_dy_Filt) -> ObjectToCenterLine_dy_Filt/1

== system PubIfDecisionTOS_MDL/TOS_20201112/TOS_2012080320/PIL_1029/ProbCalculat/ProbCalculat/ObjectProbCalculation ==
  TOS_OFMObjValid_Flag : Inport  Partition=on  PartitionDimension=1  PartitionWidth=1  PartitionOffset=0
  Object_Width : Inport  Port=2  Partition=on  PartitionDimension=1  PartitionWidth=1  PartitionOffset=0
  Object_Type : Inport  Port=3  Partition=on  PartitionDimension=1  PartitionWidth=1  PartitionOffset=0
  PIL_SameCenterLine_dyc : Inport  Port=4  Partition=on  PartitionDimension=1  PartitionWidth=1  PartitionOffset=0
  PIL_LeftCenterLine_dyc : Inport  Port=5  Partition=on  PartitionDimension=1  PartitionWidth=1  PartitionOffset=0
  PIL_RightCenterLine_dyc : Inport  Port=6  Partition=on  PartitionDimension=1  PartitionWidth=1  PartitionOffset=0
  SameLane_CoreArea_Boundary : Inport  Port=7  Partition=on  PartitionDimension=1  PartitionWidth=1  PartitionOffset=0
  SameLane_EdgeLeft_Boundary : Inport  Port=8  Partition=on  PartitionDimension=1  PartitionWidth=1  PartitionOffset=0
  SameLane_EdgeRight_Boundary : Inport  Port=9  Partition=on  PartitionDimension=1  PartitionWidth=1  PartitionOffset=0
  LeftLane_CoreArea_Boundary : Inport  Port=10  Partition=on  PartitionDimension=1  PartitionWidth=1  PartitionOffset=0
  LeftLane_EdgeLeft_Boundary : Inport  Port=11  Partition=on  PartitionDimension=1  PartitionWidth=1  PartitionOffset=0
  LeftLane_EdgeRight_Boundary : Inport  Port=12  Partition=on  PartitionDimension=1  PartitionWidth=1  PartitionOffset=0
  RightLane_CoreArea_Boundary : Inport  Port=13  Partition=on  PartitionDimension=1  PartitionWidth=1  PartitionOffset=0
  RightLane_EdgeLeft_Boundary : Inport  Port=14  Partition=on  PartitionDimension=1  PartitionWidth=1  PartitionOffset=0
  RightLane_EdgeRight_Boundary : Inport  Port=15  Partition=on  PartitionDimension=1  PartitionWidth=1  PartitionOffset=0
  Compare To Constant : simulink/Logic and Bit Operations/Compare To Constant  relop===  const=C_TOS_OFMObjIDInvilad_Val  OutDataTypeStr=boolean
      settings: AttributesFormatString=C_TOS_OFMObjIDInvilad_Val = 0
  Data Type Conversion : DataTypeConversion  OutDataTypeStr=Enum: OFM_OBJ_TYPE_E
  For Each : ForEach  DisableCoverage=on
  If : If  IfExpression=u1 ~= 0
  Merge{,1..3} (4 alike) : Merge
  ProbCalculation : Subsystem
  ProbCalculationDefault : Subsystem  TreatAsAtomicUnit=on
  "PIL_ObjLaneProb_all " : Outport  InitialOutput=0  ConcatenationDimension=1
  PIL_EgoLaneProb : Outport  Port=2  InitialOutput=0  ConcatenationDimension=1
  PIL_LeftLaneProb : Outport  Port=3  ConcatenationDimension=1
  PIL_RightLaneProb : Outport  Port=4  ConcatenationDimension=1
  wires:
  Merge2/1 -> PIL_RightLaneProb/1
  Merge1/1 -> PIL_LeftLaneProb/1
  ProbCalculationDefault/4(PIL_RightLaneProb) -> Merge2/1
  ProbCalculation/4(PIL_RightLaneProb) -> Merge2/2
  ProbCalculationDefault/3(PIL_LeftLaneProb) -> Merge1/1
  ProbCalculation/3(PIL_LeftLaneProb) -> Merge1/2
  RightLane_EdgeLeft_Boundary/1 -> ProbCalculation/13(RightLane_EdgeLeft_Boundary)
  RightLane_CoreArea_Boundary/1 -> ProbCalculation/12(RightLane_CoreArea_Boundary)
  LeftLane_EdgeRight_Boundary/1 -> ProbCalculation/11(LeftLane_EdgeRight_Boundary)
  LeftLane_EdgeLeft_Boundary/1 -> ProbCalculation/10(LeftLane_EdgeLeft_Boundary)
  LeftLane_CoreArea_Boundary/1 -> ProbCalculation/9(LeftLane_CoreArea_Boundary)
  RightLane_EdgeRight_Boundary/1 -> ProbCalculation/14(RightLane_EdgeRight_Boundary)
  PIL_RightCenterLine_dyc/1 -> ProbCalculation/5(PIL_RightCenterLine_dyc)
  PIL_LeftCenterLine_dyc/1 -> ProbCalculation/4(PIL_LeftCenterLine_dyc)
  Merge/1 -> PIL_EgoLaneProb/1
  ProbCalculationDefault/2(PIL_EgoLaneProb) -> Merge/1
  If/2 -> ProbCalculation/Action
  Compare To Constant/1 -> If/1
  If/1 -> ProbCalculationDefault/Action
  Data Type Conversion/1 -> ProbCalculation/2(Object_Type)
  ProbCalculation/2(PIL_EgoLaneProb) -> Merge/2
  SameLane_EdgeRight_Boundary/1 -> ProbCalculation/8(SameLane_EdgeRight_Boundary)
  SameLane_EdgeLeft_Boundary/1 -> ProbCalculation/7(SameLane_EdgeLeft_Boundary)
  SameLane_CoreArea_Boundary/1 -> ProbCalculation/6(SameLane_CoreArea_Boundary)
  PIL_SameCenterLine_dyc/1 -> ProbCalculation/3(PIL_SameCenterLine_dyc)
  Object_Type/1 -> Data Type Conversion/1
  Object_Width/1 -> ProbCalculation/1(Object_Width)
  TOS_OFMObjValid_Flag/1 -> Compare To Constant/1
  Merge3/1 -> "PIL_ObjLaneProb_all "/1
  ProbCalculation/1("PIL_ObjLaneProb _all ") -> Merge3/2
  ProbCalculationDefault/1("PIL_ObjLaneProb _all ") -> Merge3/1

== system PubIfDecisionTOS_MDL/TOS_20201112/TOS_2012080320/PIL_1029/ProbCalculat/ProbCalculat/Subsystem ==
  LM_SignalVerification : Inport
  Bus Creator : BusCreator  Inputs=3
  Bus Selector : BusSelector  OutputSignals=TOS_LM_LL_Bus.LM_LL_Line04.pC0,TOS_LM_LR_Bus.LM_LR_Line04.pC0,TOS_LM_RL_Bus.LM_RL_Line04.pC0,TOS_LM_RR_Bus.LM_RR_Line04.pC0
  Constant : Constant  Value=C_TOS_EgoCarWidth_Val  OutDataTypeStr=single
      settings: AttributesFormatString=C_TOS_EgoCarWidth_Val = 1.88
  EgoVehiclePro : Subsystem
  Gain : Gain  Gain=0.5  OutDataTypeStr=single
  PIL_EgoVehiclePro : Subsystem
  PIL_EgoVehicleProFilt : Outport
  wires:
  EgoVehiclePro/3(EgoVehicle_RightLaneProb) -> Bus Creator/3  "EgoVehicle_RightLaneProb"
  Gain/1 -> EgoVehiclePro/5(HalfEgoWidth)
  EgoVehiclePro/2(EgoVehicle_EgoLaneProb) -> Bus Creator/2  "EgoVehicle_EgoLaneProb"
  Bus Selector/3 -> EgoVehiclePro/3(RL_C0)  "<pC0>"
  Bus Selector/2 -> EgoVehiclePro/2(LR_C0)  "<pC0>"
  Constant/1 -> Gain/1
  LM_SignalVerification/1 -> Bus Selector/1
  Bus Selector/4 -> EgoVehiclePro/4(RR_C0)  "<pC0>"
  Bus Selector/1 -> EgoVehiclePro/1(LL_C0)  "<pC0>"
  EgoVehiclePro/1(EgoVehicle_LeftLaneProb) -> Bus Creator/1  "EgoVehicle_LeftLaneProb"
  Bus Creator/1 -> PIL_EgoVehiclePro/1(PIL_EgoVehiclePro)
  PIL_EgoVehiclePro/1(PIL_EgoVehicleProFilt) -> PIL_EgoVehicleProFilt/1  "TOS_PIL_EgoVehiclePro_bus"

== system PubIfDecisionTOS_MDL/TOS_20201112/TOS_2012080320/PIL_1029/ProbCalculat/ProbFilt/ObjinEgoLaneProb ==
  PIL_ObjinEgoLaneProb : Inport
  Demux : Demux  Outputs=80
  Mux : Mux  Inputs=80
  Prob_Filt{1..80} (80 alike) : TOS_LIB/Prob_Filt  SystemSampleTime=-1  VariantActivationTime=update diagram  Latency=0  AutoFrameSizeCalculation=off
  PIL_ObjinEgoLaneProb_Filt : Outport
  wires:
  Mux/1 -> PIL_ObjinEgoLaneProb_Filt/1
  Prob_Filt72/1 -> Mux/80  "EgoCar_LeftLaneProb"
  Prob_Filt71/1 -> Mux/79  "EgoCar_LeftLaneProb"
  Prob_Filt70/1 -> Mux/78  "EgoCar_LeftLaneProb"
  Prob_Filt69/1 -> Mux/77  "EgoCar_LeftLaneProb"
  Prob_Filt68/1 -> Mux/76  "EgoCar_LeftLaneProb"
  Prob_Filt67/1 -> Mux/75  "EgoCar_LeftLaneProb"
  Prob_Filt66/1 -> Mux/74  "EgoCar_LeftLaneProb"
  Prob_Filt80/1 -> Mux/73  "EgoCar_LeftLaneProb"
  Prob_Filt79/1 -> Mux/72  "EgoCar_LeftLaneProb"
  Prob_Filt78/1 -> Mux/71  "EgoCar_LeftLaneProb"
  Prob_Filt77/1 -> Mux/70  "EgoCar_LeftLaneProb"
  Prob_Filt76/1 -> Mux/69  "EgoCar_LeftLaneProb"
  Prob_Filt75/1 -> Mux/68  "EgoCar_LeftLaneProb"
  Prob_Filt74/1 -> Mux/67  "EgoCar_LeftLaneProb"
  Prob_Filt73/1 -> Mux/66  "EgoCar_LeftLaneProb"
  Prob_Filt65/1 -> Mux/65  "EgoCar_LeftLaneProb"
  Prob_Filt49/1 -> Mux/64  "EgoCar_LeftLaneProb"
  Prob_Filt48/1 -> Mux/63  "EgoCar_LeftLaneProb"
  Prob_Filt47/1 -> Mux/62  "EgoCar_LeftLaneProb"
  Prob_Filt46/1 -> Mux/61  "EgoCar_LeftLaneProb"
  Prob_Filt45/1 -> Mux/60  "EgoCar_LeftLaneProb"
  Prob_Filt43/1 -> Mux/59  "EgoCar_LeftLaneProb"
  Prob_Filt42/1 -> Mux/58  "EgoCar_LeftLaneProb"
  Prob_Filt58/1 -> Mux/57  "EgoCar_LeftLaneProb"
  Prob_Filt57/1 -> Mux/56  "EgoCar_LeftLaneProb"
  Prob_Filt56/1 -> Mux/55  "EgoCar_LeftLaneProb"
  Prob_Filt54/1 -> Mux/54  "EgoCar_LeftLaneProb"
  Prob_Filt53/1 -> Mux/53  "EgoCar_LeftLaneProb"
  Prob_Filt52/1 -> Mux/52  "EgoCar_LeftLaneProb"
  Prob_Filt51/1 -> Mux/51  "EgoCar_LeftLaneProb"
  Prob_Filt50/1 -> Mux/50  "EgoCar_LeftLaneProb"
  Prob_Filt41/1 -> Mux/49  "EgoCar_LeftLaneProb"
  Prob_Filt40/1 -> Mux/48  "EgoCar_LeftLaneProb"
  Prob_Filt39/1 -> Mux/47  "EgoCar_LeftLaneProb"
  Prob_Filt38/1 -> Mux/46  "EgoCar_LeftLaneProb"
  Prob_Filt37/1 -> Mux/45  "EgoCar_LeftLaneProb"
  Prob_Filt36/1 -> Mux/44  "EgoCar_LeftLaneProb"
  Prob_Filt35/1 -> Mux/43  "EgoCar_LeftLaneProb"
  Prob_Filt34/1 -> Mux/42  "EgoCar_LeftLaneProb"
  Prob_Filt64/1 -> Mux/41  "EgoCar_LeftLaneProb"
  Prob_Filt63/1 -> Mux/40  "EgoCar_LeftLaneProb"
  Prob_Filt62/1 -> Mux/39  "EgoCar_LeftLaneProb"
  Prob_Filt61/1 -> Mux/38  "EgoCar_LeftLaneProb"
  Prob_Filt60/1 -> Mux/37  "EgoCar_LeftLaneProb"
  Prob_Filt59/1 -> Mux/36  "EgoCar_LeftLaneProb"
  Prob_Filt55/1 -> Mux/35  "EgoCar_LeftLaneProb"
  Prob_Filt44/1 -> Mux/34  "EgoCar_LeftLaneProb"
  Prob_Filt33/1 -> Mux/33  "EgoCar_LeftLaneProb"
  Prob_Filt24/1 -> Mux/32  "EgoCar_LeftLaneProb"
  Prob_Filt23/1 -> Mux/31  "EgoCar_LeftLaneProb"
  Prob_Filt22/1 -> Mux/30  "EgoCar_LeftLaneProb"
  Prob_Filt21/1 -> Mux/29  "EgoCar_LeftLaneProb"
  Prob_Filt20/1 -> Mux/28  "EgoCar_LeftLaneProb"
  Prob_Filt19/1 -> Mux/27  "EgoCar_LeftLaneProb"
  Prob_Filt18/1 -> Mux/26  "EgoCar_LeftLaneProb"
  Prob_Filt32/1 -> Mux/25  "EgoCar_LeftLaneProb"
  Prob_Filt31/1 -> Mux/24  "EgoCar_LeftLaneProb"
  Prob_Filt30/1 -> Mux/23  "EgoCar_LeftLaneProb"
  Prob_Filt29/1 -> Mux/22  "EgoCar_LeftLaneProb"
  Prob_Filt28/1 -> Mux/21  "EgoCar_LeftLaneProb"
  Prob_Filt27/1 -> Mux/20  "EgoCar_LeftLaneProb"
  Prob_Filt26/1 -> Mux/19  "EgoCar_LeftLaneProb"
  Prob_Filt25/1 -> Mux/18  "EgoCar_LeftLaneProb"
  Prob_Filt17/1 -> Mux/17  "EgoCar_LeftLaneProb"
  Prob_Filt16/1 -> Mux/16  "EgoCar_LeftLaneProb"
  Prob_Filt15/1 -> Mux/15  "EgoCar_LeftLaneProb"
  Prob_Filt14/1 -> Mux/14  "EgoCar_LeftLaneProb"
  Prob_Filt13/1 -> Mux/13  "EgoCar_LeftLaneProb"
  Prob_Filt12/1 -> Mux/12  "EgoCar_LeftLaneProb"
  Prob_Filt11/1 -> Mux/11  "EgoCar_LeftLaneProb"
  Prob_Filt10/1 -> Mux/10  "EgoCar_LeftLaneProb"
  Prob_Filt9/1 -> Mux/9  "EgoCar_LeftLaneProb"
  Prob_Filt8/1 -> Mux/8  "EgoCar_LeftLaneProb"
  Prob_Filt7/1 -> Mux/7  "EgoCar_LeftLaneProb"
  Prob_Filt6/1 -> Mux/6  "EgoCar_LeftLaneProb"
  Prob_Filt5/1 -> Mux/5  "EgoCar_LeftLaneProb"
  Prob_Filt4/1 -> Mux/4  "EgoCar_LeftLaneProb"
  Prob_Filt3/1 -> Mux/3  "EgoCar_LeftLaneProb"
  Prob_Filt2/1 -> Mux/2  "EgoCar_LeftLaneProb"
  Prob_Filt1/1 -> Mux/1  "EgoCar_LeftLaneProb"
  Demux/67 -> Prob_Filt74/1
  Demux/66 -> Prob_Filt73/1
  Demux/65 -> Prob_Filt65/1
  Demux/64 -> Prob_Filt49/1
  Demux/63 -> Prob_Filt48/1
  Demux/62 -> Prob_Filt47/1
  Demux/60 -> Prob_Filt45/1
  Demux/59 -> Prob_Filt43/1
  Demux/58 -> Prob_Filt42/1
  Demux/57 -> Prob_Filt58/1
  Demux/56 -> Prob_Filt57/1
  Demux/55 -> Prob_Filt56/1
  Demux/54 -> Prob_Filt54/1
  Demux/53 -> Prob_Filt53/1
  Demux/52 -> Prob_Filt52/1
  Demux/51 -> Prob_Filt51/1
  Demux/50 -> Prob_Filt50/1
  Demux/49 -> Prob_Filt41/1
  Demux/48 -> Prob_Filt40/1
  Demux/47 -> Prob_Filt39/1
  Demux/46 -> Prob_Filt38/1
  Demux/45 -> Prob_Filt37/1
  Demux/44 -> Prob_Filt36/1
  Demux/43 -> Prob_Filt35/1
  Demux/42 -> Prob_Filt34/1
  Demux/41 -> Prob_Filt64/1
  Demux/40 -> Prob_Filt63/1
  Demux/39 -> Prob_Filt62/1
  Demux/38 -> Prob_Filt61/1
  Demux/37 -> Prob_Filt60/1
  Demux/36 -> Prob_Filt59/1
  Demux/35 -> Prob_Filt55/1
  Demux/34 -> Prob_Filt44/1
  Demux/33 -> Prob_Filt33/1
  Demux/32 -> Prob_Filt24/1
  Demux/31 -> Prob_Filt23/1
  Demux/30 -> Prob_Filt22/1
  Demux/29 -> Prob_Filt21/1
  Demux/28 -> Prob_Filt20/1
  Demux/27 -> Prob_Filt19/1
  Demux/26 -> Prob_Filt18/1
  Demux/25 -> Prob_Filt32/1
  Demux/24 -> Prob_Filt31/1
  Demux/23 -> Prob_Filt30/1
  Demux/22 -> Prob_Filt29/1
  Demux/21 -> Prob_Filt28/1
  Demux/20 -> Prob_Filt27/1
  Demux/19 -> Prob_Filt26/1
  Demux/18 -> Prob_Filt25/1
  Demux/17 -> Prob_Filt17/1
  Demux/16 -> Prob_Filt16/1
  Demux/15 -> Prob_Filt15/1
  Demux/14 -> Prob_Filt14/1
  Demux/13 -> Prob_Filt13/1
  Demux/12 -> Prob_Filt12/1
  Demux/11 -> Prob_Filt11/1
  Demux/10 -> Prob_Filt10/1
  Demux/9 -> Prob_Filt9/1
  Demux/8 -> Prob_Filt8/1
  Demux/7 -> Prob_Filt7/1
  Demux/6 -> Prob_Filt6/1
  Demux/5 -> Prob_Filt5/1
  Demux/4 -> Prob_Filt4/1
  Demux/3 -> Prob_Filt3/1
  Demux/2 -> Prob_Filt2/1
  Demux/61 -> Prob_Filt46/1
  Demux/68 -> Prob_Filt75/1
  Demux/69 -> Prob_Filt76/1
  Demux/70 -> Prob_Filt77/1
  Demux/71 -> Prob_Filt78/1
  Demux/72 -> Prob_Filt79/1
  Demux/73 -> Prob_Filt80/1
  Demux/74 -> Prob_Filt66/1
  Demux/75 -> Prob_Filt67/1
  Demux/76 -> Prob_Filt68/1
  Demux/77 -> Prob_Filt69/1
  Demux/78 -> Prob_Filt70/1
  Demux/79 -> Prob_Filt71/1
  Demux/80 -> Prob_Filt72/1
  Demux/1 -> Prob_Filt1/1
  PIL_ObjinEgoLaneProb/1 -> Demux/1
